simulink model "scenario_2_TAC_5robots_plus"  (R2020b)
settings: Solver=FixedStepAuto  StartTime=0.0  StopTime=60.0  FixedStep=1e-2  RelTol=1e-3
libraries: simulink x5
(part 2 of 2)

== matlab function scenario_2_TAC_5robots_plus/agent5/Potential_Field_controller3 ==
  data: x1 input; x2 input; agent1_x1 input; agent1_x2 input; agent2_x1 input; agent2_x2 input; agent3_x1 input; agent3_x2 input; agent4_x1 input; agent4_x2 input; L1 input; L2 input; u1 output; xa3 input; u2 output; u3 output
function [u1,u2,u3] = fcn(x1, x2, agent1_x1,agent1_x2,agent2_x1,agent2_x2,agent3_x1,agent3_x2,agent4_x1,agent4_x2,L1,L2, xa3)
coder.extrinsic('Calculate_gradient');
coder.extrinsic('Calculate_gradient_x15');
coder.extrinsic('PVF_optimizer');
coder.extrinsic('add_random');
A1=[-1,0;0,-1];
F=[2*50,2*0];
distance=sqrt((x1-90)^2+(x2-90)^2);

gradient_x=0;gradient_y=0;
agent1_gradient_x=0;agent1_gradient_y=0;
agent2_gradient_x=0;agent2_gradient_y=0;
agent3_gradient_x=0;agent3_gradient_y=0;
agent4_gradient_x=0;agent4_gradient_y=0;
[gradient_x,gradient_y]=Calculate_gradient(x1,x2,A1,F,0,30,8);
[agent1_gradient_x,agent1_gradient_y]=Calculate_gradient_dynamic(x1,x2,A1,F,agent1_x1,agent1_x2,10);
[agent2_gradient_x,agent2_gradient_y]=Calculate_gradient_dynamic(x1,x2,A1,F,agent2_x1,agent2_x2,10);
[agent3_gradient_x,agent3_gradient_y]=Calculate_gradient_dynamic(x1,x2,A1,F,agent3_x1,agent3_x2,10);
[agent4_gradient_x,agent4_gradient_y]=Calculate_gradient_dynamic(x1,x2,A1,F,agent4_x1,agent4_x2,10);
if sqrt( (x1-agent1_x1)^2+(x2-agent1_x2)^2 )<=30 %agent5 & agent1
    gradient_x=gradient_x+agent1_gradient_x;
    gradient_y=gradient_y+agent1_gradient_y;
end
if sqrt( (x1-agent2_x1)^2+(x2-agent2_x2)^2 )<=30 %agent5 & agent2
    gradient_x=gradient_x+agent2_gradient_x;
    gradient_y=gradient_y+agent2_gradient_y;
end
if sqrt( (x1-agent3_x1)^2+(x2-agent3_x2)^2 )<=30 %agent5 & agent3
    gradient_x=gradient_x+agent3_gradient_x;
    gradient_y=gradient_y+agent3_gradient_y;
end
if sqrt( (x1-agent4_x1)^2+(x2-agent4_x2)^2 )<=30 %agent5 & agent4
    gradient_x=gradient_x+agent4_gradient_x;
    gradient_y=gradient_y+agent4_gradient_y;
end
gradient_x=gradient_x;
gradient_y=gradient_y;
gradient_z=0;

Gradient_all=[gradient_x;gradient_y;gradient_z];
Li=0.2;
Bi=[0,cos(pi/6),-cos(pi/6);
    -1,sin(pi/6),sin(pi/6);
    Li,Li,Li;];

R1=[cos(xa3),-sin(xa3),0;
    sin(xa3),cos(xa3),0;
    0,0,1;];
R=0.02;
gx=R1*inv(Bi')*R;
A=Gradient_all'*gx;

%H=[1];
%H=[1,0;0,1];
%H=[0,0,0;0,0,0;0,0,0];
% H=[1,0,0;0,1,0;0,0,1];
 H=(1/2)*gx'*gx;
b=[0];
F=[-2*gx'*40*Gradient_all];
%=[];
u1=0;u2=0;u3=0;
U=PVF_optimizer(H,b,A,F,distance,gradient_x,gradient_y);

u1=U(1,1);
u2=U(2,1);
u3=U(3,1);

== matlab function scenario_2_TAC_5robots_plus/agent5/STL_barrier 1 ==
  data: b output; b50 output; b1 output; b2 output; yita output; h output; t input; p1 input; p2 input; L1 input; L2 input; yita50 output; h50 output; agent1_x1 input; agent1_x2 input; agent2_x1 input; agent2_x2 input; agent3_x1 input; agent3_x2 input; agent4_x1 input; agent4_x2 input
function [b,b50,b1,b2,yita,h,yita50,h50] = fcn(t,p1,p2,L1,L2, agent1_x1,agent1_x2,agent2_x1,agent2_x2,agent3_x1,agent3_x2,agent4_x1,agent4_x2)
d1=L1;
d2=L2;

d11=50;
d22=0;

d111=0;d222=30;

b=25*exp(-0.32*t)+5-sqrt( (p1-d1)^2 + (p2-d2)^2 ); %STL_tracking
yita=-25*exp(-0.32*t)+10;
h=15-sqrt( (p1-d1)^2 + (p2-d2)^2 );


b50=125*exp(-0.07*(t))+5-sqrt( (p1-d11)^2 + (p2-d22)^2 );%STL_visiting 
yita50=-125*exp(-0.07*(t))+5;
h50=10-sqrt( (p1-d11)^2 + (p2-d22)^2 );


% b50=5-sqrt( (p1-d11)^2 + (p2-d22)^2 );
% yita50=5;
% h50=10-sqrt( (p1-d11)^2 + (p2-d22)^2 );

b1=sqrt( (p1-d11)^2 + (p2-d22)^2 )-0;%STL_visiting_trigger

b21=sqrt( (p1-d111)^2 + (p2-d222)^2 )-6;
b5_1=sqrt( (p1-agent1_x1)^2 + (p2-agent1_x2)^2 )-10;
b5_2=sqrt( (p1-agent2_x1)^2 + (p2-agent2_x2)^2 )-10;
b5_3=sqrt( (p1-agent3_x1)^2 + (p2-agent3_x2)^2 )-10;
b5_4=sqrt( (p1-agent4_x1)^2 + (p2-agent4_x2)^2 )-10;
% b22=sqrt( (p1-agent5_x1)^2 + (p2-agent5_x2)^2 )-6;
b2=-(1/20)*log(exp(-20*b21)+exp(-20*b5_1)+exp(-20*b5_2)+exp(-20*b5_3)+exp(-20*b5_4)); %obstacle_avoidence_trigger

== matlab function scenario_2_TAC_5robots_plus/agent5/STL_controller1_visiting ==
  data: x1 input; x2 input; L1 input; L2 input; b_in input; u1 output; xa3 input; u2 output; u3 output; t input
function [u1,u2,u3]= fcn(x1, x2,L1,L2, b_in, xa3,t)
coder.extrinsic('quadoptimizer');
%coder.extrinsic('save');
d1=50; d2=0;

partial_b=(1/2)*((x1-d1)^2+(x2-d2)^2)^(-1/2);
partial_b_x=[-2*partial_b*(x1-d1),-2*partial_b*(x2-d2),0];


Li=0.2;
Bi=[0,cos(pi/6),-cos(pi/6);
    -1,sin(pi/6),sin(pi/6);
    Li,Li,Li;];

R1=[cos(xa3),-sin(xa3),0;
    sin(xa3),cos(xa3),0;
    0,0,1;];
R=0.02;

gx=R1*inv(Bi')*R;

A=partial_b_x*gx;

H=[1,0,0;0,1,0;0,0,1];
%H=[1];

b=5*b_in-0.07*125*exp(-0.07*(t))-10;

%  b=500*b_in-50;


u1=0;u2=0;u3=0;
U=quadoptimizer(H,b,A);

%U=quadprod(H,[],-A,b);

u1=U(1,1);
u2=U(2,1);
u3=U(3,1);

== matlab function scenario_2_TAC_5robots_plus/agent5/STL_controller_tracking1 ==
  data: x1 input; x2 input; L1 input; L2 input; b_in input; u1 output; xa3 input; u2 output; u3 output; t input
function [u1,u2,u3]= fcn(x1, x2,L1,L2, b_in, xa3,t)
coder.extrinsic('quadoptimizer');
%coder.extrinsic('save');
d1=L1; d2=L2;

partial_b=(1/2)*((x1-d1)^2+(x2-d2)^2)^(-1/2);
partial_b_x=[-2*partial_b*(x1-d1),-2*partial_b*(x2-d2),0];
partial_b_L=[2*partial_b*(x1-d1),2*partial_b*(x2-d2)];
pho1=sqrt(partial_b_L(1,1)^2+partial_b_L(1,2)^2);
Li=0.2;
Bi=[0,cos(pi/6),-cos(pi/6);
    -1,sin(pi/6),sin(pi/6);
    Li,Li,Li;];

R1=[cos(xa3),-sin(xa3),0;
    sin(xa3),cos(xa3),0;
    0,0,1;];
R=0.02;

gx=R1*inv(Bi')*R;

A=partial_b_x*gx;

H=[1,0,0;0,1,0;0,0,1];
%H=[1];

% b=200*b_in-0.37*25*exp(-0.37*t)-300-30*pho1;
b=200*b_in-0.32*25*exp(-0.32*t)-300-30*pho1;


u1=0;u2=0;u3=0;
U=quadoptimizer(H,b,A);

%U=quadprod(H,[],-A,b);

u1=U(1,1);
u2=U(2,1);
u3=U(3,1);

== matlab function scenario_2_TAC_5robots_plus/agent5/leader1 ==
  data: t input; L1 output; L2 output
function [L1,L2] = fcn(t)
L1=-30*sin(1*t);
L2=-30*cos(1*t);

== matlab function scenario_2_TAC_5robots_plus/agent1/MATLAB Function2 ==
  data: x1 input; theta output; y1 input
function theta = fcn(x1, y1)
theta=atan2(y1,x1);

== matlab function scenario_2_TAC_5robots_plus/agent1/Potential_Field_controller3 ==
  data: x1 input; x2 input; agent2_x1 input; agent2_x2 input; agent3_x1 input; agent3_x2 input; agent4_x1 input; agent4_x2 input; agent5_x1 input; agent5_x2 input; L1 input; L2 input; u1 output; xa3 input; u2 output; u3 output
function [u1,u2,u3] = fcn(x1, x2, agent2_x1,agent2_x2,agent3_x1,agent3_x2,agent4_x1,agent4_x2,agent5_x1,agent5_x2,L1,L2, xa3)
coder.extrinsic('Calculate_gradient');
coder.extrinsic('Calculate_gradient_dynamic');
coder.extrinsic('Calculate_gradient_x15');
coder.extrinsic('PVF_optimizer');
coder.extrinsic('add_random');
A1=[-1,0;0,-1];
F=[2*L1,2*L2];
distance=sqrt((x1-90)^2+(x2-90)^2);

gradient_x=0;gradient_y=0;
agent2_gradient_x=0;agent2_gradient_y=0;
agent3_gradient_x=0;agent3_gradient_y=0;
agent4_gradient_x=0;agent4_gradient_y=0;
agent5_gradient_x=0;agent5_gradient_y=0;
[gradient_x,gradient_y]=Calculate_gradient(x1,x2,A1,F,0,30,8);
[agent2_gradient_x,agent2_gradient_y]=Calculate_gradient_dynamic(x1,x2,A1,F,agent2_x1,agent2_x2,10);
[agent3_gradient_x,agent3_gradient_y]=Calculate_gradient_dynamic(x1,x2,A1,F,agent3_x1,agent3_x2,10);
[agent4_gradient_x,agent4_gradient_y]=Calculate_gradient_dynamic(x1,x2,A1,F,agent4_x1,agent4_x2,10);
[agent5_gradient_x,agent5_gradient_y]=Calculate_gradient_dynamic(x1,x2,A1,F,agent5_x1,agent5_x2,10);
if sqrt( (x1-agent2_x1)^2+(x2-agent2_x2)^2 )<=30 %agent1 & agent2
    gradient_x=gradient_x+agent2_gradient_x;
    gradient_y=gradient_y+agent2_gradient_y;
end
if sqrt( (x1-agent3_x1)^2+(x2-agent3_x2)^2 )<=30 %agent1 & agent3
    gradient_x=gradient_x+agent3_gradient_x;
    gradient_y=gradient_y+agent3_gradient_y;
end
if sqrt( (x1-agent4_x1)^2+(x2-agent4_x2)^2 )<=30 %agent1 & agent4
    gradient_x=gradient_x+agent4_gradient_x;
    gradient_y=gradient_y+agent4_gradient_y;
end
if sqrt( (x1-agent5_x1)^2+(x2-agent5_x2)^2 )<=30 %agent1 & agent5
    gradient_x=gradient_x+agent5_gradient_x;
    gradient_y=gradient_y+agent5_gradient_y;
end
gradient_x=gradient_x;
gradient_y=gradient_y;
    

% gradient_x=Gradient(1,1);
% gradient_y=Gradient(1,2);
gradient_z=0;

Gradient_all=[gradient_x;gradient_y;gradient_z];
Li=0.2;
Bi=[0,cos(pi/6),-cos(pi/6);
    -1,sin(pi/6),sin(pi/6);
    Li,Li,Li;];

R1=[cos(xa3),-sin(xa3),0;
    sin(xa3),cos(xa3),0;
    0,0,1;];
R=0.02;
gx=R1*inv(Bi')*R;
A=Gradient_all'*gx;

%H=[1];
%H=[1,0;0,1];
%H=[0,0,0;0,0,0;0,0,0];
% H=[1,0,0;0,1,0;0,0,1];
 H=(1/2)*gx'*gx;
b=[0];
F=[-2*gx'*40*Gradient_all];
%=[];
u1=0;u2=0;u3=0;
U=PVF_optimizer(H,b,A,F,distance,gradient_x,gradient_y);

u1=U(1,1);
u2=U(2,1);
u3=U(3,1);

== matlab function scenario_2_TAC_5robots_plus/agent1/STL_barrier 1 ==
  data: b output; b50 output; b1 output; b2 output; yita output; h output; t input; p1 input; p2 input; L1 input; L2 input; yita50 output; h50 output; agent2_x1 input; agent2_x2 input; agent3_x1 input; agent3_x2 input; agent4_x1 input; agent4_x2 input; agent5_x1 input; agent5_x2 input
function [b,b50,b1,b2,yita,h,yita50,h50] = fcn(t,p1,p2,L1,L2,agent2_x1,agent2_x2,agent3_x1,agent3_x2,agent4_x1,agent4_x2,agent5_x1,agent5_x2)
d1=L1;
d2=L2;

d11=50;
d22=0;

d111=0;d222=30;

b=25*exp(-0.32*t)+5-sqrt( (p1-d1)^2 + (p2-d2)^2 ); %STL_tracking
yita=-25*exp(-0.32*t)+10;
h=15-sqrt( (p1-d1)^2 + (p2-d2)^2 );


b50=60*exp(-0.125*(t))+5-sqrt( (p1-d11)^2 + (p2-d22)^2 );%STL_visiting 
yita50=-60*exp(-0.125*(t))+5;
h50=10-sqrt( (p1-d11)^2 + (p2-d22)^2 );


% b50=5-sqrt( (p1-d11)^2 + (p2-d22)^2 );
% yita50=5;
% h50=10-sqrt( (p1-d11)^2 + (p2-d22)^2 );

b1=sqrt( (p1-d11)^2 + (p2-d22)^2 )-0;%STL_visiting_trigger

b21=sqrt( (p1-d111)^2 + (p2-d222)^2 )-6;
b1_2=sqrt( (p1-agent2_x1)^2 + (p2-agent2_x2)^2 )-10;
b1_3=sqrt( (p1-agent3_x1)^2 + (p2-agent3_x2)^2 )-10;
b1_4=sqrt( (p1-agent4_x1)^2 + (p2-agent4_x2)^2 )-10;
b1_5=sqrt( (p1-agent5_x1)^2 + (p2-agent5_x2)^2 )-10;
b2=-(1/20)*log(exp(-20*b21) + exp(-20*b1_2)+ exp(-20*b1_3)+ exp(-20*b1_4)+ exp(-20*b1_5)); %obstacle_avoidence_trigger

== matlab function scenario_2_TAC_5robots_plus/agent1/STL_controller1_visiting ==
  data: x1 input; x2 input; L1 input; L2 input; b_in input; u1 output; xa3 input; u2 output; u3 output; t input
function [u1,u2,u3]= fcn(x1, x2,L1,L2, b_in, xa3,t)
coder.extrinsic('quadoptimizer');
%coder.extrinsic('save');
d1=50; d2=0;

partial_b=(1/2)*((x1-d1)^2+(x2-d2)^2)^(-1/2);
partial_b_x=[-2*partial_b*(x1-d1),-2*partial_b*(x2-d2),0];


Li=0.2;
Bi=[0,cos(pi/6),-cos(pi/6);
    -1,sin(pi/6),sin(pi/6);
    Li,Li,Li;];

R1=[cos(xa3),-sin(xa3),0;
    sin(xa3),cos(xa3),0;
    0,0,1;];
R=0.02;

gx=R1*inv(Bi')*R;

A=partial_b_x*gx;

H=[1,0,0;0,1,0;0,0,1];
%H=[1];

b=300*b_in-0.125*60*exp(-0.125*(t))-50;

%  b=500*b_in-50;


u1=0;u2=0;u3=0;
U=quadoptimizer(H,b,A);

%U=quadprod(H,[],-A,b);

u1=U(1,1);
u2=U(2,1);
u3=U(3,1);

== matlab function scenario_2_TAC_5robots_plus/agent1/STL_controller_tracking1 ==
  data: x1 input; x2 input; L1 input; L2 input; b_in input; u1 output; xa3 input; u2 output; u3 output; t input
function [u1,u2,u3]= fcn(x1, x2,L1,L2, b_in, xa3,t)
coder.extrinsic('quadoptimizer');
%coder.extrinsic('save');
d1=L1; d2=L2;

partial_b=(1/2)*((x1-d1)^2+(x2-d2)^2)^(-1/2);
partial_b_x=[-2*partial_b*(x1-d1),-2*partial_b*(x2-d2),0];
partial_b_L=[2*partial_b*(x1-d1),2*partial_b*(x2-d2)];
pho1=sqrt(partial_b_L(1,1)^2+partial_b_L(1,2)^2);
Li=0.2;
Bi=[0,cos(pi/6),-cos(pi/6);
    -1,sin(pi/6),sin(pi/6);
    Li,Li,Li;];

R1=[cos(xa3),-sin(xa3),0;
    sin(xa3),cos(xa3),0;
    0,0,1;];
R=0.02;

gx=R1*inv(Bi')*R;

A=partial_b_x*gx;

H=[1,0,0;0,1,0;0,0,1];
%H=[1];

% b=200*b_in-0.37*25*exp(-0.37*t)-300-30*pho1;
b=200*b_in-0.32*25*exp(-0.32*t)-300-30*pho1;


u1=0;u2=0;u3=0;
U=quadoptimizer(H,b,A);

%U=quadprod(H,[],-A,b);

u1=U(1,1);
u2=U(2,1);
u3=U(3,1);

== matlab function scenario_2_TAC_5robots_plus/agent2/STL_barrier 1 ==
  data: b output; b50 output; b1 output; b2 output; yita output; h output; t input; p1 input; p2 input; L1 input; L2 input; yita50 output; h50 output; agent1_x1 input; agent1_x2 input; agent3_x1 input; agent3_x2 input; agent4_x1 input; agent4_x2 input; agent5_x1 input; agent5_x2 input
function [b,b50,b1,b2,yita,h,yita50,h50] = fcn(t,p1,p2,L1,L2,agent1_x1,agent1_x2,agent3_x1,agent3_x2,agent4_x1,agent4_x2,agent5_x1,agent5_x2)
d1=L1;
d2=L2;

d11=50;
d22=0;

d111=0;d222=30;

b=25*exp(-0.32*t)+5-sqrt( (p1-d1)^2 + (p2-d2)^2 ); %STL_tracking
yita=-25*exp(-0.32*t)+10;
h=15-sqrt( (p1-d1)^2 + (p2-d2)^2 );


b50=60*exp(-0.125*(t))+5-sqrt( (p1-d11)^2 + (p2-d22)^2 );%STL_visiting 
yita50=-60*exp(-0.125*(t))+5;
h50=10-sqrt( (p1-d11)^2 + (p2-d22)^2 );


% b50=5-sqrt( (p1-d11)^2 + (p2-d22)^2 );
% yita50=5;
% h50=10-sqrt( (p1-d11)^2 + (p2-d22)^2 );

b1=sqrt( (p1-d11)^2 + (p2-d22)^2 )-0;%STL_visiting_trigger

b21=sqrt( (p1-d111)^2 + (p2-d222)^2 )-6;
b2_1=sqrt( (p1-agent1_x1)^2 + (p2-agent1_x2)^2 )-10;
b2_3=sqrt( (p1-agent3_x1)^2 + (p2-agent3_x2)^2 )-10;
b2_4=sqrt( (p1-agent4_x1)^2 + (p2-agent4_x2)^2 )-10;
b2_5=sqrt( (p1-agent5_x1)^2 + (p2-agent5_x2)^2 )-10;
% b22=sqrt( (p1-agent5_x1)^2 + (p2-agent5_x2)^2 )-6;
b2=-(1/20)*log(exp(-20*b21)+exp(-20*b2_1)+exp(-20*b2_3)+exp(-20*b2_4)+exp(-20*b2_5)); %obstacle_avoidence_trigger

== matlab function scenario_2_TAC_5robots_plus/agent1/leader1 ==
  data: t input; L1 output; L2 output
function [L1,L2] = fcn(t)
L1=30*sin(1*t);
L2=30*cos(1*t);

== matlab function scenario_2_TAC_5robots_plus/agent1/omnidirectional robot1 ==
  data: ua1 input; xa1_dot output; ua2 input; ua3 input; xa3 input; xa2_dot output; xa3_dot output
function [xa1_dot,xa2_dot,xa3_dot]= fcn(ua1,ua2,ua3,xa3)

Li=0.2;
Bi=[0,cos(pi/6),-cos(pi/6);
    -1,sin(pi/6),sin(pi/6);
    Li,Li,Li;];

R1=[cos(xa3),-sin(xa3),0;
    sin(xa3),cos(xa3),0;
    0,0,1;];
R=0.02;

A=R1*inv(Bi')*R*[ua1;ua2;ua3];
xa1_dot=A(1,1);
xa2_dot=A(2,1);
xa3_dot=A(3,1);

== matlab function scenario_2_TAC_5robots_plus/agent1/regulation function  ==
  data: STL_u1 input; U1 output; STL_u2 input; STL_u3 input; STLv_u1 input; STLv_u2 input; STLv_u3 input; obs_u1 input; obs_u2 input; obs_u3 input; b1 input; U2 output; U3 output; b2 input
function [U1,U2,U3] = fcn(STL_u1,STL_u2,STL_u3,STLv_u1,STLv_u2,STLv_u3,obs_u1,obs_u2,obs_u3,b1,b2)
U_track=[STL_u1;STL_u2;STL_u3];
U_visit=[STLv_u1;STLv_u2;STLv_u3];
U_obs=[obs_u1;obs_u2;obs_u3];

k=0.065;
lambda=1-exp(-k*max(b1,0));
U_goal=lambda*U_track+(1-lambda)*U_visit;
% U_goal=[0;0;0];
% U_goal=U_track;
j=0.15;
gamma=1-exp(-j*max(b2,0));
U=gamma*U_goal+(1-gamma)*U_obs;

% U=U_goal;
U1=0;U2=0;U3=0;
U1=U(1,1);
U2=U(2,1);
U3=U(3,1);

== matlab function scenario_2_TAC_5robots_plus/agent1/velocity_constraint1 ==
  data: U1 input; Uc1 output; U2 input; U3 input; xa3 input; v_max input; Uc2 output; Uc3 output
function [Uc1,Uc2,Uc3] = fcn(U1,U2,U3,xa3,v_max)

Li=0.2;
Bi=[0,cos(pi/6),-cos(pi/6);
    -1,sin(pi/6),sin(pi/6);
    Li,Li,Li;];

R1=[cos(xa3),-sin(xa3),0;
    sin(xa3),cos(xa3),0;
    0,0,1;];
R=0.02;
gx=R1*inv(Bi')*R;

U=[U1;U2;U3];
V=[0;0;0];
V=gx*U;
if V(1,1)^2+V(2,1)^2<=v_max^2
     U(1,1)= U(1,1);
     U(2,1)= U(2,1);
else 
    U(1,1)=sqrt(v_max^2/(V(1,1)^2+V(2,1)^2))*U(1,1);
    U(2,1)=sqrt(v_max^2/(V(1,1)^2+V(2,1)^2))*U(2,1);
    U(3,1)=sqrt(v_max^2/(V(1,1)^2+V(2,1)^2))*U(3,1);
end

Uc1=U(1,1);
Uc2=U(2,1);
Uc3=U(3,1);

== matlab function scenario_2_TAC_5robots_plus/agent5/omnidirectional robot1 ==
  data: ua1 input; xa1_dot output; ua2 input; ua3 input; xa3 input; xa2_dot output; xa3_dot output
function [xa1_dot,xa2_dot,xa3_dot]= fcn(ua1,ua2,ua3,xa3)

Li=0.2;
Bi=[0,cos(pi/6),-cos(pi/6);
    -1,sin(pi/6),sin(pi/6);
    Li,Li,Li;];

R1=[cos(xa3),-sin(xa3),0;
    sin(xa3),cos(xa3),0;
    0,0,1;];
R=0.02;

A=R1*inv(Bi')*R*[ua1;ua2;ua3];
xa1_dot=A(1,1);
xa2_dot=A(2,1);
xa3_dot=A(3,1);

== matlab function scenario_2_TAC_5robots_plus/agent5/regulation function  ==
  data: STL_u1 input; U1 output; STL_u2 input; STL_u3 input; STLv_u1 input; STLv_u2 input; STLv_u3 input; obs_u1 input; obs_u2 input; obs_u3 input; b1 input; U2 output; U3 output; b2 input
function [U1,U2,U3] = fcn(STL_u1,STL_u2,STL_u3,STLv_u1,STLv_u2,STLv_u3,obs_u1,obs_u2,obs_u3,b1,b2)
U_track=[STL_u1;STL_u2;STL_u3];
U_visit=[STLv_u1;STLv_u2;STLv_u3];
U_obs=[obs_u1;obs_u2;obs_u3];

k=0.065;
% lambda=1-exp(-k*max(b1,0));
lambda=0;
U_goal=lambda*U_track+(1-lambda)*U_visit;
% U_goal=[0;0;0];
% U_goal=U_track;
j=0.15;
gamma=1-exp(-j*max(b2,0));
U=gamma*U_goal+(1-gamma)*U_obs;

% U=U_goal;
U1=0;U2=0;U3=0;
U1=U(1,1);
U2=U(2,1);
U3=U(3,1);

== matlab function scenario_2_TAC_5robots_plus/agent5/velocity_constraint1 ==
  data: U1 input; Uc1 output; U2 input; U3 input; xa3 input; v_max input; Uc2 output; Uc3 output
function [Uc1,Uc2,Uc3] = fcn(U1,U2,U3,xa3,v_max)

Li=0.2;
Bi=[0,cos(pi/6),-cos(pi/6);
    -1,sin(pi/6),sin(pi/6);
    Li,Li,Li;];

R1=[cos(xa3),-sin(xa3),0;
    sin(xa3),cos(xa3),0;
    0,0,1;];
R=0.02;
gx=R1*inv(Bi')*R;

U=[U1;U2;U3];
V=[0;0;0];
V=gx*U;
if V(1,1)^2+V(2,1)^2<=v_max^2
     U(1,1)= U(1,1);
     U(2,1)= U(2,1);
else 
    U(1,1)=sqrt(v_max^2/(V(1,1)^2+V(2,1)^2))*U(1,1);
    U(2,1)=sqrt(v_max^2/(V(1,1)^2+V(2,1)^2))*U(2,1);
    U(3,1)=sqrt(v_max^2/(V(1,1)^2+V(2,1)^2))*U(3,1);
end

Uc1=U(1,1);
Uc2=U(2,1);
Uc3=U(3,1);

== matlab function scenario_2_TAC_5robots_plus/agent2/STL_controller1_visiting ==
  data: x1 input; x2 input; L1 input; L2 input; b_in input; u1 output; xa3 input; u2 output; u3 output; t input
function [u1,u2,u3]= fcn(x1, x2,L1,L2, b_in, xa3,t)
coder.extrinsic('quadoptimizer');
%coder.extrinsic('save');
d1=50; d2=0;

partial_b=(1/2)*((x1-d1)^2+(x2-d2)^2)^(-1/2);
partial_b_x=[-2*partial_b*(x1-d1),-2*partial_b*(x2-d2),0];


Li=0.2;
Bi=[0,cos(pi/6),-cos(pi/6);
    -1,sin(pi/6),sin(pi/6);
    Li,Li,Li;];

R1=[cos(xa3),-sin(xa3),0;
    sin(xa3),cos(xa3),0;
    0,0,1;];
R=0.02;

gx=R1*inv(Bi')*R;

A=partial_b_x*gx;

H=[1,0,0;0,1,0;0,0,1];
%H=[1];

b=300*b_in-0.125*60*exp(-0.125*(t))-50;

%  b=500*b_in-50;


u1=0;u2=0;u3=0;
U=quadoptimizer(H,b,A);

%U=quadprod(H,[],-A,b);

u1=U(1,1);
u2=U(2,1);
u3=U(3,1);
